simulink model "quadraticmodel"  (R2020a)
settings: Solver=VariableStepAuto  StartTime=0.0  StopTime=10.0  RelTol=1e-3
undefined symbols (not defined in the file or in its folder): k, m, q
libraries: simulink x1
settings Model: Creator=User  LastModifiedBy=User

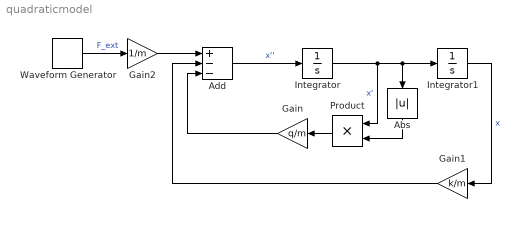
== system quadraticmodel ==
  Abs : Abs
  Add : Sum  Inputs=+--
  Gain : Gain  Gain=q/m
  Gain1 : Gain  Gain=k/m
  Gain2 : Gain  Gain=1/m
  Integrator : Integrator
  Integrator1 : Integrator
  Product : Product
  Waveform Generator : simulink/Sources/Waveform Generator  OutMin=[]  OutMax=[]  OutDataTypeStr=double  SelectedSignal=1  BlockNames=MultiportSwitch_e3df3653d217406  SampleTime=0.1
  wires:
  Integrator/1 -> Abs/1, Integrator1/1, Product/1  "x'"
  Integrator1/1 -> Gain1/1  "x"
  Add/1 -> Integrator/1  "x''"
  Abs/1 -> Product/2
  Product/1 -> Gain/1
  Gain2/1 -> Add/1
  Waveform Generator/1 -> Gain2/1  "F_ext"
  Gain/1 -> Add/3
  Gain1/1 -> Add/2
